simulink model "polyphase_clock_sync_HDL_2019"  (R2019b)
settings: Solver=FixedStepAuto  StartTime=0.0  StopTime=10e-3  FixedStep=1e-6  RelTol=1e-3
undefined symbols (not defined in the file or in its folder): image, port_label
libraries: aldec_ahdl x2, commfilt2 x2, commchan3 x1, commrandsrc3 x1, simulink_extras x1, dspsrcs4 x1, commdigbbndpm3 x1, simulink x1, hdlsllib x1, commsync2 x1, dspsigops x1
settings Model: ald_sampling=[1e-3,5,1e-6,4,0,0,0]  ald_sim_cfg={0,0,0,0,'',0,'C:\Users\student_1\Desktop\Sokołowski_praca_dyplomowa\My_design\polyphase_clock_sync.aws',1,0,0}  ald_log_cfg={'$(model_name)',0,'3',0,'$(model_name).log',1,15}  ald_macros={0,'',0,'',0,''}  ald_scripts={'','','',''}  ald_dlg_cfg={'12.0',0}  Creator=student_1  LastModifiedBy=thomas
settings DebuggingCC: SFMachineParentedDataDiag=error

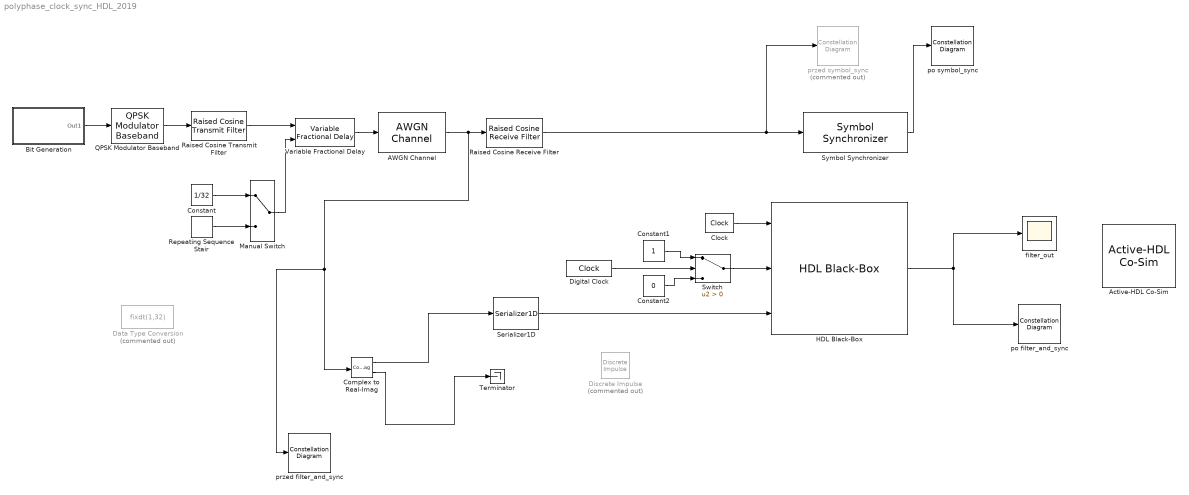
== system polyphase_clock_sync_HDL_2019 ==
  AWGN Channel : commchan3/AWGN Channel  InputProcessing=Columns as channels (frame based)  seed=67  noiseMode="Signal to noise ratio  (SNR)"  EbNodB=10  EsNodB=10  SNRdB=100  bitsPerSym=1  Ps=1/2  Tsym=1  variance=1
  Active-HDL Co-Sim : aldec_ahdl/Active-HDL Co-Sim  Tag=Active-HDL_Co-Sim_close  hdl_period=1  hdl_tscale=us  sys_period=[1, 0]  sys_tscale=As In Simulator  wav_fn=$(model_name)  wav_settings=[0,3]  sim_cfg=[0,0,0]  dbg=off  auto_start=off  gen_tb=[0,1,15]  batch_sim=off  tb_fn=$(model_name).log  metavalue_map=[0,0]  sim_resolution=[1,0,0]  active_page=0  aws_en=off  ahdl_en=off  blk_ver=10.5a.RTM  macro_en=[0,0,0]
      settings: SourceProductName=Active-HDL Toolbox
  Bit Generation : Subsystem
      mask Display: disp('Bit Frame\nGeneration')
  Clock : simulink_extras/Flip Flops/Clock  period=10e-6
  Complex to Real-Imag : ComplexToRealImag
  Constant : Constant  Value=1/32
  Constant1 : Constant
  Constant2 : Constant  Value=0
  Data Type Conversion : DataTypeConversion  Commented=on  OutMin=-1024  OutMax=1024  OutDataTypeStr=fixdt(1,32)
  Digital Clock : DigitalClock  SampleTime=1e-6
  Discrete Impulse : dspsrcs4/Discrete  Impulse  Commented=on  Delay=1  SampleTime=1  FrameSample=1  OutputFrames=off  dataType=double  isSigned=on  wordLen=16  udDataType=sfix(16)  fracBitsMode=Best precision  numFracBits=15  OutDataTypeStr=double  LastOutDataTypeStr=double
  HDL Black-Box : aldec_ahdl/HDL Black-Box  Tag=Active-HDL_BB_lib  module_m=polyphase_clock_sync  ports_cfg={CLK,0,1,2,0,Inherited,8,0,0,0,0,0}{ARESTN,0,1,2,0,Inherited,8,0,0,0,0,0}{DIN,0,-1,2,0,Inherited,0,0,0,0,0,0}{DOUT,1,-1,2,0,1,0,0,0,0,0,0}  params={CHANNELS,32,INTEGER}{DATA_WIDTH,32,INTEGER}{FACTOR_WIDTH,12,INTEGER}{AXIS_DATA_WIDTH,32,INTEGER}{SAMPLES_PER_SYMBOL,2,INTEGER}{OVERSAMPLING_RATE,32,INTEGER}  block_mask=image('HDLBlackBox.jpg','center'); disp('polyphase_clock_sync');port_label('input', 1, 'CLK');port_label('input', 2, 'ARESTN');port_label('input', 3, 'DIN');port_label('output', 1, 'DOUT');  config=[3,1]  inp=[3, 8, 1, 0, 0, 0, 2, 8, 1, 0, 0, 0, 2, 0, abs(32-1 - 0) + 1, 0, 0, 0, 2]  out=[1, 0, abs(32-1 - 0) + 1, 0, 0, 0, 2]  sampling=[1, -1, -1, -1, 1]  active_page={774,476,5,{0,{80,0,0,1},{35,1,2,1},{65,2,2,1},{70,3,2,1},{70,4,2,1},{60,5,2,1},{60,6,2,1},{50,7,2,1},{35,8,2,1},{35,9,2,1},{119,10,0,1}},{1,{106,0,0,1},{55,1,2,1},{70,2,2,1},{75,3,2,1},{75,4,2,1},{45,5,2,1},{45,6,2,1},{45,7,2,1},{165,8,0,1}},{2,{120,0,0,1},{100,1,2,1},{190,2,2,1},{100,3,2,1},{120,4,0,1}},{3,{94,0,0,1},{58,1,2,1},{58,2,2,1},{70,3,2,1},{58,4,2,1}},{4,{83,0,0,1},{70,1,2,1},{80,2,2,1},{50,3,2,1},{50,4,2,1}},{5,{125,0,0,1},{330,1,2,1},{220,2,2,1}},{6,{95,0,0,1},{95,1,1,1},{70,2,2,1},{50,3,1,1},{80,4,1,1},{35,5,2,1},{35,6,2,1},{65,7,0,1},{150,8,0,1}}}  param_val={32,-1,32,-1,12,-1,32,-1,2,-1,32,-1}  clk_val=[0]  ce_val=[0]  blk_ver=10.5a.RTM  blk_conf=0  user_conv=0
      settings: SourceProductName=Active-HDL Toolbox
  Manual Switch : ManualSwitch
  QPSK Modulator Baseband : commdigbbndpm3/QPSK Modulator Baseband  InType=Bit  Enc=Gray  Ph=pi/4  outDtype=double  outWordLen=16  outUDDataType=sfix(16)  outFracLenMode=Best precision  outFracLen=15  outDataTypeStr=double  outLastDataTypeStr=double
  Raised Cosine Receive Filter : commfilt2/Raised Cosine Receive Filter  filtType=Square root  R=0.4  filtSpan=10  N=2  downFactor=1  downOffset=0  filterGain=1  InputProcessing=Columns as channels (frame based)  RateOptions=Enforce single-rate processing  framing=Mute  checkCoeff=off  variableName=rcRxFilt  currentFiltSpan=10  D=5  inputOffset=0  sampMode=Mute  saveAsFlag=0  rateMode=Downsampling  checkGain=Normalized  launchFVT=on  roundingMode=Floor  overflowMode=off  coeffDataTypeStr=Inherit: Same word length as input  coeffMin=[]  coeffMax=[]  coeffLastDataTypeStr=Inherit: Same word length as input  accumDataTypeStr=Inherit: Same as product output  accumLastDataTypeStr=Inherit: Same as product output  outputDataTypeStr=Inherit: Same as accumulator  outputMin=[]  outputMax=[]  outputLastDataTypeStr=Inherit: Same as accumulator
  Raised Cosine Transmit Filter : commfilt2/Raised Cosine Transmit Filter  filtType=Square root  R=0.4  filtSpan=10  N=2  filterGain=1  InputProcessing=Columns as channels (frame based)  RateOptions=Enforce single-rate processing  framing=Mute  checkCoeff=off  variableName=rcTxFilt  checkGain=Normalized  sampMode=Mute  saveAsFlag=0  currentFiltSpan=10  D=(10)/2  launchFVT=on  roundingMode=Floor  overflowMode=off  coeffDataTypeStr=Inherit: Same word length as input  coeffMin=[]  coeffMax=[]  coeffLastDataTypeStr=Inherit: Same word length as input  outputDataTypeStr=Inherit: Same as accumulator  outputMin=[]  outputMax=[]  outputLastDataTypeStr=Inherit: Same as accumulator
  Repeating Sequence Stair : simulink/Sources/Repeating Sequence Stair  OutValues=[(1:1:31)/32 (31:-1:1)/32]  tsamp=-1  OutMin=[]  OutMax=[]  OutDataTypeStr=double  OutputDataTypeScalingMode=double  OutDataType=fixdt(0,8)  ConRadixGroup=Best Precision: Vector-wise  OutScaling=2^-12
  Serializer1D : hdlsllib/HDL Operations/Serializer1D  Ratio=1000  IdleCycles=0  validIn=off  startOut=off  validOut=off  inputDataDimensions=-1  inputSampleTime=-1  inputSignalType=auto
      settings: SourceProductBaseCode=SL
  Switch : Switch  Criteria=u2 > Threshold
  Symbol Synchronizer : commsync2/Symbol Synchronizer  Modulation=PAM/PSK/QAM  TimingErrorDetector=Zero-Crossing (decision-directed)  SamplesPerSymbol=2  DampingFactor=sqrt(2)/2  NormalizedLoopBandwidth=0.01  DetectorGain=2.7  TimingErrorOutputPort=off  SimulateUsing=Code generation
      settings: SourceProductBaseCode=CM
  Terminator : Terminator
  Variable Fractional Delay : dspsigops/Variable Fractional Delay  mode=OBSOLETE  modeActive=Linear  L=4  FarrowL=4  R=10  alpha=1  dmax=400  InputProcessing=Columns as channels (frame based)  ic=0  noDFT=off  fallbackFIR=Clip to the minimum value necessary for centered kernel  fallbackFarrow=Clip to the minimum value necessary for centered kernel  roundingMode=Zero  overflowMode=off
      settings: SourceProductBaseCode=DS
  filter_out : Scope
  po filter_and_sync : ConstellationDiagram
  po symbol_sync : ConstellationDiagram
  przed filter_and_sync : ConstellationDiagram
  przed symbol_sync : ConstellationDiagram  Commented=on
  wires:
  Bit Generation/1(Out1) -> QPSK Modulator Baseband/1
  QPSK Modulator Baseband/1 -> Raised Cosine Transmit Filter/1
  Constant/1 -> Manual Switch/1
  Manual Switch/1 -> Variable Fractional Delay/2
  Repeating Sequence Stair/1 -> Manual Switch/2
  Variable Fractional Delay/1 -> AWGN Channel/1
  Raised Cosine Transmit Filter/1 -> Variable Fractional Delay/1
  HDL Black-Box/1 -> filter_out/1, po filter_and_sync/1
  AWGN Channel/1 -> przed filter_and_sync/1, Complex to Real-Imag/1, Raised Cosine Receive Filter/1
  Raised Cosine Receive Filter/1 -> przed symbol_sync/1, Symbol Synchronizer/1
  Symbol Synchronizer/1 -> po symbol_sync/1
  Switch/1 -> HDL Black-Box/2
  Clock/1 -> HDL Black-Box/1
  Complex to Real-Imag/1 -> Serializer1D/1
  Complex to Real-Imag/2 -> Terminator/1
  Constant2/1 -> Switch/3
  Constant1/1 -> Switch/1
  Digital Clock/1 -> Switch/2
  Serializer1D/1 -> HDL Black-Box/3

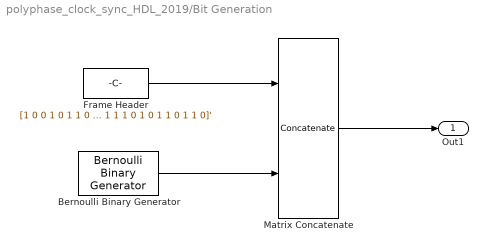
== system polyphase_clock_sync_HDL_2019/Bit Generation ==
  Bernoulli Binary Generator : commrandsrc3/Bernoulli Binary Generator  ProbabilityOfZero=0.5  SeedSource=Parameter  Seed=61  SampleTime=1  SamplesPerFrame=960  OutputDataType=double  SimulateUsing=Interpreted execution
  Frame Header : Constant  Value=[1 0 0 1 0 1 1 0 1 1 1 0 1 0 1 1 0 1 1 0 1 0 0 1 0 1 1 0 1 1 1 0 1 0 1 1 0 1 1 0]'  VectorParams1D=off  OutDataTypeStr=double  SampleTime=10e-3
  Matrix Concatenate : Concatenate  Mode=Multidimensional array
  Out1 : Outport  VectorParamsAs1DForOutWhenUnconnected=off
  wires:
  Matrix Concatenate/1 -> Out1/1
  Frame Header/1 -> Matrix Concatenate/1
  Bernoulli Binary Generator/1 -> Matrix Concatenate/2
